simulink model "tank_model"  (R2022b)
settings: Solver=VariableStepAuto  StartTime=0.0  StopTime=st  RelTol=1e-3
model workspace (MAT data in the model file):
  estimator = ss
  estimator.IOSize_ = [3 7]
  estimator.Data_ = ltipack.ssdata
  estimator.Data_.a = [0.994575478083  -4.00386186307e-05  4.00372173094e-05; 4.00386186307e-05  0.990886301562  0; -4.00372173094e-05  0  0.979001899996]
  estimator.Data_.b = [0.008804225352  -0.00230110435336  -3.74217459475e-19  1.15459632451e-17  0.00638498286454  4.00386186307e-05  -4.00372173094e-05; 0.000200273144639  0.00220102131548  0.00490237726859  -1.62693118453e-17  0  0.0100841690399  0; -0.000210270637514  -0.00220094426854  0.00190085525656  0.0210094528356  0  0  0.0218985051252]
  estimator.Data_.c = [1  0  0; 0  1  0; 0  0  1]
  estimator.Data_.d = [0  0  0  0  0  0  0; 0  0  0  0  0  0  0; 0  0  0  0  0  0  0]
  estimator.Data_.Delay.Input = [0; 0; 0; 0; 0; 0; 0]
  estimator.Data_.Delay.Output = [0; 0; 0]
  estimator.Data_.Delay.Internal = []
  estimator.Data_.Ts = 0
values from neighbouring files (symbols this model uses):
  Ad = expm(A*T)    [intialise_tank_model.m]
  Ad2 = Ad - K2d*C    [intialise_tank_model.m]
  AU_Info = zeros(9,1)    [intialise_tank_model.m]    (also in tank_model_config.m = [)
  AY_Info = zeros(9,1)    [intialise_tank_model.m]    (also in tank_model_config.m = [)
  Bd = pinv(A)*(Ad - eye(3))*B    [intialise_tank_model.m]
  Bd2 = [Bd K2d]    [intialise_tank_model.m]
  C = eye(3)    [intialise_tank_model.m]
  D_Info = [1;5;3;3]    [intialise_tank_model.m]    (also in tank_model_config.m = [)
  in = [-0.05, 0.05, randi(1000)]    [intialise_tank_model.m]    (also in tank_model_config.m = [)
  intialStates = [10; 15; 20]    [intialise_tank_model.m]    (also in tank_model_config.m = [)
  intialStates2 = [9.5; 14.5; 19.5]    [intialise_tank_model.m]    (also in tank_model_config.m = [)
  mn = [-0.15, 0.15, randi(1000)]    [intialise_tank_model.m]    (also in tank_model_config.m = [)
undefined symbols (not defined in the file or in its folder): k
settings Model: Creator=matth  LastModifiedBy=matth

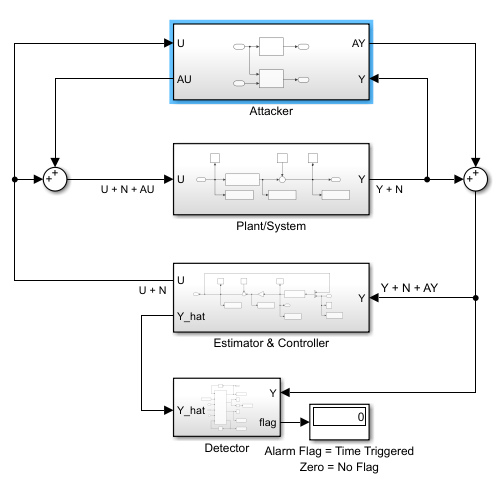
[thumbnail: Simulink's stored preview of the top-level diagram]
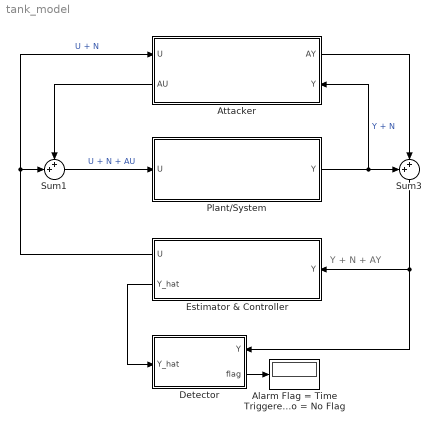
== system tank_model ==
  note: Y + N + AY
  Alarm Flag = Time Triggered Zero = No Flag : Display
      settings: Format=binary (Stored Integer)  Decimation=3
  Attacker : Subsystem
      settings: PortSchema="{\"entries\":[{\"content\":{\"sides\":[{\"content\":{\"connectorIds\":[\"In1\",\"Out2\"]},\"type\":\"ConnectorPlacement.EquallySpacedRectSide\",\"uuid\":\"4d2c954e-3783-4521-af26-8a82cc4b32cd\"},{\"content\":{\"connectorIds\":[\"Out1\",\"In2\"],\"side\":\"RIGHT\"},\"type\":\"ConnectorPlacement.EquallySpacedRectSide\",\"uuid\":\"20497f4c-c211-46bf-96cd-185fe78a9b68\"},{\"content\":{\"connectorIds\":[],\"side\":\"TOP\"},\"type\":\"ConnectorPlacement.EquallySpacedRectSide\",\"uuid\":\"c1c38c65-2dff-4c6b-8fd3-2db485026c68\"}]},\"type\":\"ConnectorPlacement.EquallySpacedConnector\",\"uuid\":\"f8362177-d8ac-417c-bb01-70017971ff65\"}],\"packageUris\":[\"http://schema.mathworks.com/mf0/Connector/R2020b\"],\"version\":\"1.0\"}"
  Detector : Subsystem
      settings: PortSchema="{\"entries\":[{\"content\":{\"sides\":[{\"content\":{\"connectorIds\":[\"In1\"]},\"type\":\"ConnectorPlacement.EquallySpacedRectSide\",\"uuid\":\"811fb41d-5a12-4eec-833e-d49a5c2e282b\"},{\"content\":{\"connectorIds\":[\"In2\",\"Out1\"],\"side\":\"RIGHT\"},\"type\":\"ConnectorPlacement.EquallySpacedRectSide\",\"uuid\":\"04d53c4c-6d2b-4acd-89bb-14f15194261a\"},{\"content\":{\"connectorIds\":[],\"side\":\"TOP\"},\"type\":\"ConnectorPlacement.EquallySpacedRectSide\",\"uuid\":\"89dc32ec-b9ce-412c-b0d2-757c8eabdfac\"}]},\"type\":\"ConnectorPlacement.EquallySpacedConnector\",\"uuid\":\"473bd4bb-9f4b-4b39-9d8b-388edab30c43\"}],\"packageUris\":[\"http://schema.mathworks.com/mf0/Connector/R2020b\"],\"version\":\"1.0\"}"
  Estimator & Controller : Subsystem
  Plant/System : Subsystem
  Sum1 : Sum  Inputs=++|
  Sum3 : Sum  Inputs=++|
  wires:
  Sum1/1 -> Plant/System/1(U)  "U + N + AU"
  Detector/1(flag) -> Alarm Flag = Time Triggered Zero = No Flag/1
  Sum3/1 -> Detector/2(Y), Estimator & Controller/1(Y)
  Plant/System/1(Y) -> Sum3/1, Attacker/2(Y)  "Y + N"
  Estimator & Controller/1(U) -> Attacker/1(U), Sum1/2  "U + N"
  Estimator & Controller/2(Y_hat) -> Detector/1(Y_hat)
  Attacker/2(AU) -> Sum1/1
  Attacker/1(AY) -> Sum3/2

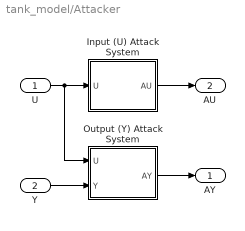
== system tank_model/Attacker ==
  U : Inport
  Y : Inport  Port=2
  Input (U) Attack System : Subsystem
  Output (Y) Attack System : Subsystem
  AY : Outport
  AU : Outport  Port=2
  wires:
  Output (Y) Attack System/1(AY) -> AY/1
  Y/1 -> Output (Y) Attack System/2(Y)
  U/1 -> Output (Y) Attack System/1(U), Input (U) Attack System/1(U)
  Input (U) Attack System/1(AU) -> AU/1

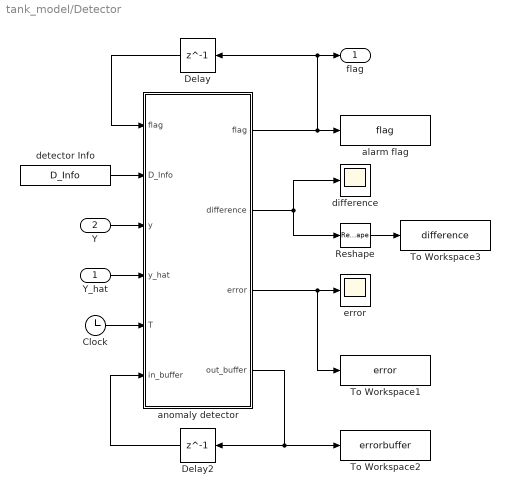
== system tank_model/Detector ==
  Y_hat : Inport
  Y : Inport  Port=2
  Clock : Clock
  Delay : Delay  DelayLength=1  InitialCondition=0
  Delay2 : Delay  DelayLength=1  InitialCondition=0
  Reshape : Reshape
  To Workspace1 : ToWorkspace  VariableName=error  SampleTime=-1
  To Workspace2 : ToWorkspace  VariableName=errorbuffer  SampleTime=-1
  To Workspace3 : ToWorkspace  VariableName=difference  SampleTime=-1
  alarm flag : ToWorkspace  VariableName=flag  SampleTime=-1
  anomaly detector : MATLAB Function  TreatAsAtomicUnit=on
  detector Info : Constant  Value=D_Info
  difference : Scope
  error : Scope
  flag : Outport
  wires:
  Y_hat/1 -> anomaly detector/4(y_hat)
  Delay/1 -> anomaly detector/1("flag ")
  anomaly detector/1(flag) -> alarm flag/1, flag/1, Delay/1
  Clock/1 -> anomaly detector/5(T)
  anomaly detector/3(error) -> To Workspace1/1, error/1
  Y/1 -> anomaly detector/3(y)
  anomaly detector/2(difference) -> Reshape/1, difference/1
  detector Info/1 -> anomaly detector/2(D_Info)
  Delay2/1 -> anomaly detector/6(in_buffer)
  anomaly detector/4(out_buffer) -> To Workspace2/1, Delay2/1
  Reshape/1 -> To Workspace3/1

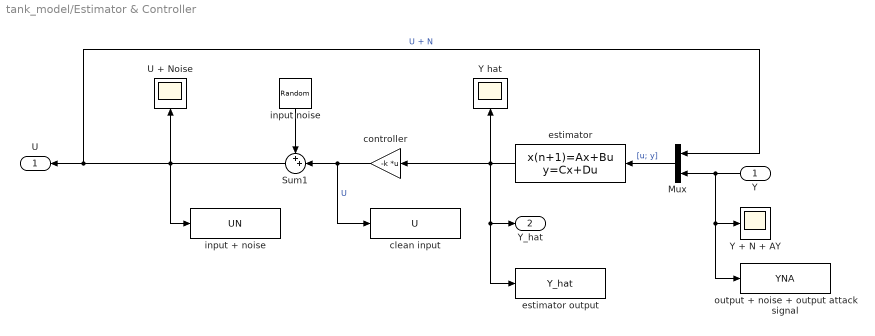
== system tank_model/Estimator & Controller ==
  Y : Inport
  Mux : Mux  Inputs=2
  Sum1 : Sum  Inputs=++|
  U + Noise : Scope
  Y + N + AY : Scope
  Y hat : Scope
  clean input : ToWorkspace  VariableName=U  SampleTime=-1
  controller : Gain  Gain=-k  Multiplication=Matrix(K*u)
  estimator : DiscreteStateSpace  A=Ad2  B=Bd2  C=C  D=Bd2*0  InitialCondition=intialStates2  SampleTime=-1
  estimator output : ToWorkspace  VariableName=Y_hat  SampleTime=-1
  input + noise : ToWorkspace  VariableName=UN  SampleTime=-1
  input noise : UniformRandomNumber  Minimum=in(1)  Maximum=in(2)  Seed=in(3)  SampleTime=0.01
  output + noise + output attack signal : ToWorkspace  VariableName=YNA  SampleTime=-1
  U : Outport
  Y_hat : Outport  Port=2
  wires:
  input noise/1 -> Sum1/1
  estimator/1 -> Y hat/1, controller/1, estimator output/1, Y_hat/1
  Sum1/1 -> Mux/1, U/1, input + noise/1, U + Noise/1  "U + N"
  controller/1 -> Sum1/2, clean input/1  "U"
  Mux/1 -> estimator/1  "[u; y]"
  Y/1 -> output + noise + output attack signal/1, Y + N + AY/1, Mux/2

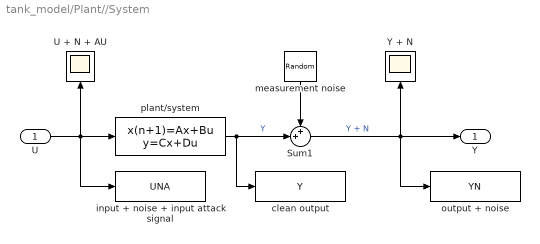
== system tank_model/Plant//System ==
  U : Inport
  Sum1 : Sum  Inputs=++|
  U + N + AU : Scope
  Y + N : Scope
  clean output : ToWorkspace  VariableName=Y  SampleTime=-1
  input + noise + input attack signal : ToWorkspace  VariableName=UNA  SampleTime=-1
  measurement noise : UniformRandomNumber  Minimum=mn(1)  Maximum=mn(2)  Seed=mn(3)  SampleTime=0.01
  output + noise : ToWorkspace  VariableName=YN  SampleTime=-1
  plant/system : DiscreteStateSpace  A=Ad  B=Bd  C=C  D=Bd*0  InitialCondition=intialStates  SampleTime=-1
  Y : Outport
  wires:
  plant/system/1 -> clean output/1, Sum1/2  "Y"
  measurement noise/1 -> Sum1/1
  U/1 -> U + N + AU/1, input + noise + input attack signal/1, plant/system/1
  Sum1/1 -> Y/1, output + noise/1, Y + N/1  "Y + N"

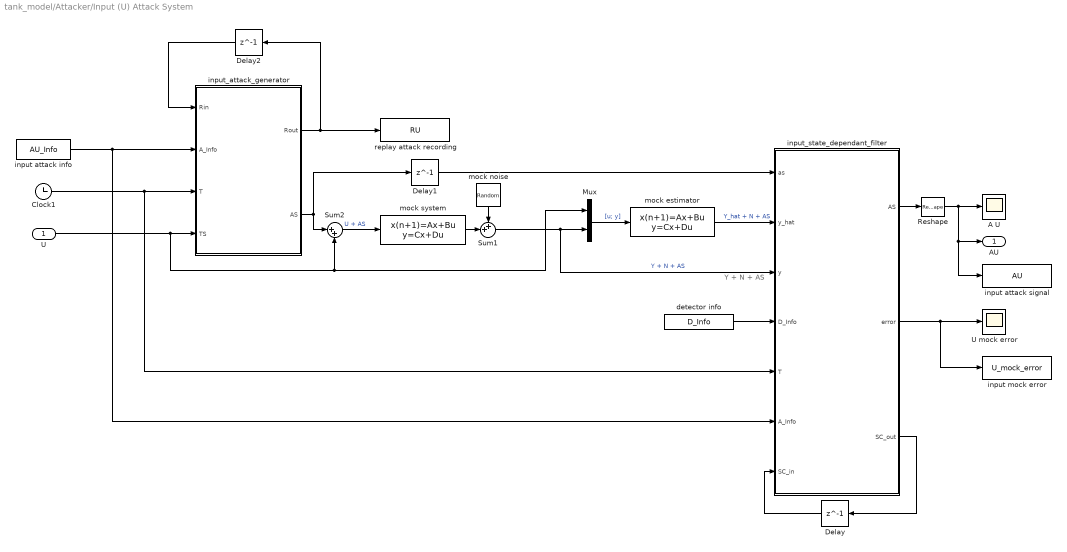
== system tank_model/Attacker/Input (U) Attack System ==
  note: Y + N + AS
  U : Inport
  A U : Scope
  Clock1 : Clock
  Delay : Delay  DelayLength=1
  Delay1 : Delay  DelayLength=1
  Delay2 : Delay  DelayLength=1  InitialCondition=zeros(100,4);
  Mux : Mux  Inputs=2
  Reshape : Reshape
  Sum1 : Sum  Inputs=++|
  Sum2 : Sum  Inputs=|++
  U mock error : Scope
  detector info : Constant  Value=D_Info
  input attack info : Constant  Value=AU_Info
  input attack signal : ToWorkspace  VariableName=AU  SampleTime=-1
  input mock error : ToWorkspace  VariableName=U_mock_error  SampleTime=-1
  input_attack_generator : MATLAB Function  TreatAsAtomicUnit=on
  input_state_dependant_filter : MATLAB Function  TreatAsAtomicUnit=on
  mock estimator : DiscreteStateSpace  A=Ad2  B=Bd2  C=C  D=Bd2*0  InitialCondition=intialStates2  SampleTime=-1
  mock noise : UniformRandomNumber  Minimum=mn(1)  Maximum=mn(2)  Seed=mn(3)  SampleTime=0.01
  mock system : DiscreteStateSpace  A=Ad  B=Bd  C=C  D=Bd*0  InitialCondition=intialStates  SampleTime=1/100
  replay attack recording : ToWorkspace  VariableName=RU  SampleTime=-1
  AU : Outport
  wires:
  Clock1/1 -> input_attack_generator/3(T), input_state_dependant_filter/5(T)
  input_attack_generator/2(AS) -> Sum2/1, Delay1/1
  input attack info/1 -> input_attack_generator/2(A_Info), input_state_dependant_filter/6(A_Info)
  Mux/1 -> mock estimator/1  "[u; y]"
  detector info/1 -> input_state_dependant_filter/4(D_Info)
  mock estimator/1 -> input_state_dependant_filter/2(y_hat)  "Y_hat + N + AS"
  input_state_dependant_filter/3(SC_out) -> Delay/1
  Delay/1 -> input_state_dependant_filter/7(SC_in)
  Sum1/1 -> input_state_dependant_filter/3(y), Mux/2  "Y + N + AS"
  input_state_dependant_filter/2(error) -> U mock error/1, input mock error/1
  mock system/1 -> Sum1/2
  mock noise/1 -> Sum1/1
  Sum2/1 -> mock system/1  "U + AS"
  input_attack_generator/1(Rout) -> Delay2/1, replay attack recording/1
  Delay2/1 -> input_attack_generator/1(Rin)
  input_state_dependant_filter/1(AS) -> Reshape/1
  Reshape/1 -> A U/1, AU/1, input attack signal/1
  U/1 -> Mux/1, Sum2/2, input_attack_generator/4(TS)
  Delay1/1 -> input_state_dependant_filter/1(as)

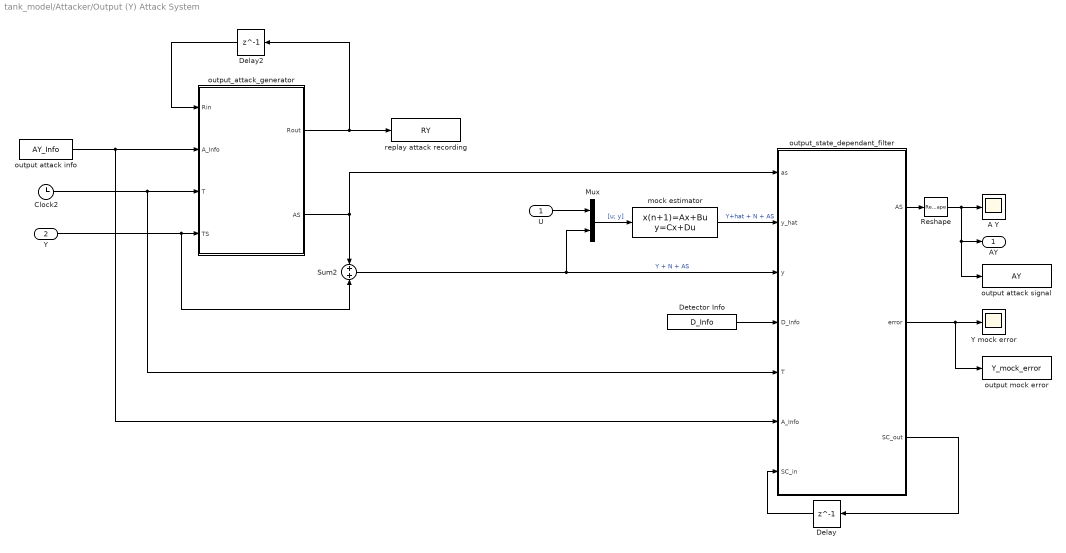
== system tank_model/Attacker/Output (Y) Attack System ==
  U : Inport
  Y : Inport  Port=2
  A Y : Scope
  Clock2 : Clock
  Delay : Delay  DelayLength=1
  Delay2 : Delay  DelayLength=1  InitialCondition=zeros(100,3);
  Detector Info : Constant  Value=D_Info
  Mux : Mux  Inputs=2
  Reshape : Reshape
  Sum2 : Sum  Inputs=+|+
  Y mock error : Scope
  mock estimator : DiscreteStateSpace  A=Ad2  B=Bd2  C=C  D=Bd2*0  InitialCondition=intialStates2  SampleTime=1/100
  output attack info : Constant  Value=AY_Info
  output attack signal : ToWorkspace  VariableName=AY  SampleTime=-1
  output mock error : ToWorkspace  VariableName=Y_mock_error  SampleTime=-1
  output_attack_generator : MATLAB Function  TreatAsAtomicUnit=on
  output_state_dependant_filter : MATLAB Function  TreatAsAtomicUnit=on
  replay attack recording : ToWorkspace  VariableName=RY  SampleTime=-1
  AY : Outport
  wires:
  output_state_dependant_filter/2(error) -> Y mock error/1, output mock error/1
  Delay/1 -> output_state_dependant_filter/7(SC_in)
  mock estimator/1 -> output_state_dependant_filter/2(y_hat)  "Y+hat + N + AS"
  Clock2/1 -> output_state_dependant_filter/5(T), output_attack_generator/3(T)
  Detector Info/1 -> output_state_dependant_filter/4(D_Info)
  output_state_dependant_filter/3(SC_out) -> Delay/1
  Mux/1 -> mock estimator/1  "[u; y]"
  output attack info/1 -> output_state_dependant_filter/6(A_Info), output_attack_generator/2(A_Info)
  output_attack_generator/2(AS) -> output_state_dependant_filter/1(as), Sum2/1
  U/1 -> Mux/1
  Sum2/1 -> Mux/2, output_state_dependant_filter/3(y)  "Y + N + AS"
  Y/1 -> Sum2/2, output_attack_generator/4(TS)
  Delay2/1 -> output_attack_generator/1(Rin)
  output_attack_generator/1(Rout) -> Delay2/1, replay attack recording/1
  Reshape/1 -> output attack signal/1, AY/1, A Y/1
  output_state_dependant_filter/1(AS) -> Reshape/1

== matlab function tank_model/Attacker/Output (Y) Attack System/output_state_dependant_filter ==
  data: as input; y_hat input; y input; D_Info input; T input; A_Info input; AS output; error output; SC_in input; SC_out output
% Matthew Reaney, QUB
% April 2023
% https://github.com/mattr862/three-tank-water-system

function [AS, error, SC_out] = Y_state_dependant_filter(as, y_hat, y, D_Info, T, A_Info,  SC_in)
%outputs = Attack Signal, error, Succcessful stealthy attack Count Out
%inputs = Attack Signal, Y_hat, Y, detector info, time, attack info,  Succcessful stealthy attack Count In
AS = zeros(3,1); % intialize attack signal

if A_Info(7) ~= 0
    %% Stealthy Attack Enabled
    % Succcessful stealthy attack Count (SC)
    if T == 0
        SC_in = 0;
    end
    SC_out = SC_in;

    % Stealty success console output
    if T == A_Info(6)
        fprintf('\nInput: Successfully preformed %i stealthy attacks out of a possible %.2i\n', int16(SC_out), int16((A_Info(6) - A_Info(5))*100)); 
    end
    
    % Mock Detector Responce
    difference = (y - y_hat);
    error = norm(difference, Inf);
    
    %If signal is stealthy use it
    if error < D_Info(1) && T >= A_Info(5) && T <= A_Info(6)
        AS = as;
        SC_out = SC_in + 1;
    end

else
    %% Stealthy Attack disabled
    AS = as;
    error = 0;
    SC_out = 0;
end

== matlab function tank_model/Detector/anomaly detector ==
  data: flag input; flag output; D_Info input; y input; y_hat input; T input; in_buffer input; difference output; error output; out_buffer output
% Matthew Reaney, QUB
% April 2023
% https://github.com/mattr862/three-tank-water-system

function [flag, difference, error, out_buffer] = detector(flag, D_Info, y, y_hat, T, in_buffer)
%% prevent flags during intialising system
if T < 0.25 
    flag = 0;
    difference = y - y_hat;
    error = norm(difference, Inf);
    in_buffer = zeros(100,1);
    out_buffer = in_buffer;
    out_buffer(1) = error;
else
    %% Calculate error/flag status for current iteration
    difference = y - y_hat; %difference between x and x^
    error = norm(difference, Inf); %absolute of infinity norm of error
    
    %% Store error in buffer
    out_buffer = in_buffer;
    out_buffer(1) = error;
    for i = 1:99
         out_buffer(i+1) = in_buffer(i);
         i = i + 1;
    end

    %% Evaluating error in buffer
    if flag == 0
        if D_Info(2) > 1 && D_Info(3) > 1 && D_Info(4) > 1
            % calculate number of consecutive errors exceeding the threshold
            consecutive = 0; i = 0;
            for i = 1:D_Info(3)
                if  out_buffer(i) >= D_Info(1)
                    consecutive = consecutive + 1;
                end
                i = i + 1;
            end
            if consecutive >= D_Info(3) && flag == 0 % consecutive errors check 
                flag = T;
                fprintf(['\nAnomaly detector flag raised at %f\n' ...
                    'Due to sufficent consecutive errors exceeding the threshold\n'], T);
            end
            
            % calculate number of total errors exceeding the threshold
            total = 0; i = 0;
            for i = 1:D_Info(2)
                if  out_buffer(i) >= D_Info(1)
                    total = total + 1;
                end
                i = i + 1;
            end
            if total >= D_Info(4) && flag == 0 % total errors check
                flag = T;
                fprintf(['\nAnomaly detector flag raised at %f\n' ...
                    'Due to sufficent total errors exceeding the threshold\n'], T);
            end
        else
            if error >= D_Info(1)
                flag = T;
                fprintf('\nAnomaly detector flag raised at %f\n', T);
                fprintf('Error Value = %f\n', error);
            end
        end
    end
end

== matlab function tank_model/Attacker/Input (U) Attack System/input_state_dependant_filter ==
  data: AS output; as input; y_hat input; y input; D_Info input; T input; A_Info input; error output; SC_in input; SC_out output
% Matthew Reaney, QUB
% April 2023
% https://github.com/mattr862/three-tank-water-system

function [AS, error, SC_out] = U_state_dependant_filter(as, y_hat, y, D_Info, T, A_Info,  SC_in)
%outputs = Attack Signal, error, Succcessful stealthy attack Count Out
%inputs = Attack Signal, Y_hat, Y, detector info, time, attack info,  Succcessful stealthy attack Count In
AS = zeros(4,1); % intialize attack signal

if A_Info(7) ~= 0
    %% Stealthy Attack Enabled
    % Succcessful stealthy attack Count (SC)
    if T == 0
        SC_in = 0;
    end
    SC_out = SC_in;

    % Stealty success console output
    if T == A_Info(6)
        fprintf('\nInput: Successfully preformed %i stealthy attacks out of a possible %.2i\n', int16(SC_out), int16((A_Info(6) - A_Info(5))*100)); 
    end
    
    % Mock Detector Responce
    difference = (y - y_hat);
    error = norm(difference, Inf);
    
    %If signal is stealthy use it
    if error < D_Info(1) && T >= A_Info(5) && T <= A_Info(6)
        AS = as;
        SC_out = SC_in + 1;
    end

else
    %% Stealthy Attack disabled
    AS = as;
    error = 0;
    SC_out = 0;
end

== matlab function tank_model/Attacker/Input (U) Attack System/input_attack_generator ==
  settings: updateMethod=DISCRETE
  data: Rout output; Rin input; A_Info input; T input; TS input; AS output
% Matthew Reaney, QUB
% April 2023
% https://github.com/mattr862/three-tank-water-system

function [Rout, AS] = U_attack_generator(Rin, A_Info, T, TS) 
%outputs = Recording Outout, Attack Signal
%inputs = Recording input, attack info, time, target signal
AS = zeros(4,1); % intialize attack signal

%% Replay attack buffer
if T == 0
    Rin = zeros(100, 4);
    Rout = Rin;
    Rout(1,:) = transpose(TS);
else
    Rout = Rin;
    Rout(1,:) = transpose(TS);
    for i = 1:99
         Rout(i+1,:) = Rin(i,:);
         i = i + 1;
    end
end

%% Attack Modeling
if T >= A_Info(5) && T <= A_Info(6) % attack time period
    i = 1;
    for i = 1:4
        switch A_Info(i)
            case 1 % FDI
                AS(i) = A_Info(8)*rand(1);
            case 2 % Bias
                AS(i) = A_Info(9); 
            case 3 % Dos
                AS(i) = -TS(i);
            case 4 % Sign_alt
                AS(i) = -2*TS(i);
            case 5 % Rerouting
                TSR = [TS(3); TS(4); TS(1); TS(2)]; % swaps values
                AS(i) = -TS(i) + TSR(i); % Combine with blank signal
            case 6 % Replay
                ti = uint16((A_Info(6)-A_Info(5))*100); % convert time to index value
                AS(i) = -TS(i) + Rin(ti,i);                
            otherwise % None
                AS(i) = 0;
        end
        i = i + 1;
    end
end      

%% Console output
if T == 0 && (A_Info(1) ~= 0 || A_Info(2) ~= 0 || A_Info(3) ~= 0 || A_Info(4) ~= 0) 
    if A_Info(7) == 1
        fprintf('Attempting Stealthy Attacks on Input from %f to %.2f\n', A_Info(5), A_Info(6));
    else
        fprintf('Attacking on Input from %f to %.2f\n', A_Info(5), A_Info(6));
    end
    i = 1;
    for i = 1:4
        switch A_Info(i)
            case 1 % FDI
                fprintf('Input %i: FDI Attack\n', int8(i));
            case 2 % Bias
                fprintf('Input %i: Bias Attack\n', int8(i));
            case 3 % Dos
                fprintf('Input %i: Dos Attack\n', int8(i));
            case 4 % Sign_alt
                fprintf('Input %i: Sign_alt Attack\n', int8(i));
            case 5 % Rerouting
                fprintf('Input %i: Rerouting Attack\n', int8(i));
            case 6 % Replay
                fprintf('Input %i: Replay Attack\n', int8(i));
                if A_Info(5)-(A_Info(6)-A_Info(5)) < 0
                    fprintf('Warning: Not enough time to record for replay attack duration\n');
                end
            otherwise
        end
        i = i + 1;
    end
end

== matlab function tank_model/Attacker/Output (Y) Attack System/output_attack_generator ==
  settings: updateMethod=DISCRETE
  data: Rout output; Rin input; A_Info input; T input; TS input; AS output
% Matthew Reaney, QUB
% April 2023
% https://github.com/mattr862/three-tank-water-system

function [Rout, AS] = Y_attack_generator(Rin, A_Info, T, TS) 
%outputs = Recording Outout, Attack Signal
%inputs = Recording input, attack info, time, target signal
AS = zeros(3,1); % intialize attack signal

%% Replay attack buffer
if T == 0
    Rin = zeros(100, 3);
    Rout = Rin;
    Rout(1,:) = transpose(TS);
else
    Rout = Rin;
    Rout(1,:) = transpose(TS);
    for i = 1:99
         Rout(i+1,:) = Rin(i,:);
         i = i + 1;
    end
end

%% Attack Modeling
if T >= A_Info(5) && T <= A_Info(6) % attack time period
    i = 1;
    for i = 1:3
        switch A_Info(i)
            case 1 % FDI
                AS(i) = A_Info(8)*rand(1);
            case 2 % Bias
                AS(i) = A_Info(9); 
            case 3 % Dos
                AS(i) = -TS(i);
            case 4 % Sign_alt
                AS(i) = -2*TS(i); 
            case 5 % Rerouting
                TSR = [TS(2); TS(1); TS(3)]; % swaps values
                AS(i) = -TS(i) + TSR(i); % Combine with blank signal
            case 6 % Replay
                ti = uint16((A_Info(6)-A_Info(5))*100); % convert time to index value
                AS(i) = -TS(i) + Rin(ti,i);
            otherwise % None
                AS(i) = 0;
        end
        i = i + 1;
    end
end      

%% Console output
if T == 0 && (A_Info(1) ~= 0 || A_Info(2) ~= 0 || A_Info(3) ~= 0)
    if A_Info(7) == 1
        fprintf('Attempting Stealthy Attacks on Output from %f to %.2f\n', A_Info(5), A_Info(6));
    else
        fprintf('Attacking Output from %f to %.2f\n', A_Info(5), A_Info(6));
    end
    i = 1;
    for i = 1:3
        switch A_Info(i)
            case 1 % FDI
                fprintf('Output %i: FDI Attack\n', int8(i));
            case 2 % Bias
                fprintf('Output %i: Bias Attack\n', int8(i));
            case 3 % Dos
                fprintf('Output %i: Dos Attack\n', int8(i));
            case 4 % Sign_alt
                fprintf('Output %i: Sign_alt Attack\n', int8(i));
            case 5 % Rerouting
                fprintf('Output %i: Rerouting Attack\n', int8(i));
            case 6 % Replay
                fprintf('Output %i: Replay Attack\n', int8(i));
                if A_Info(5)-(A_Info(6)-A_Info(5)) < 0
                    fprintf('Warning: Not enough time to record for replay attack duration\n');
                end
            otherwise
        end
        i = i + 1;
    end
end
